simulink model "c00014M_harness"  (R2018a)
settings: Solver=ode3  StartTime=0.0  StopTime=10.0  RelTol=1e-3  EnableMultiTasking=on
undefined symbols (not defined in the file): b, DiscIntNeverNeededParam, J, K, L, PosMinimaW4, R, sigbuilder_block
(part 11 of 46)

== system c00014M_harness/M018/Cyber ==
  note: Sensors
  note: Inputs For Window1
  note: Inputs for Window 2
  note: Inputs for window 3
  note: Inputs for window 4
  note: Users
  note: Users
  note: Sensors
  note: Users
  note: Sensors
  note: Users
  note: Sensors
  note: USERS
      | ---------------------------------
      | 0: None
      | 1: Ventana Arriba
      | 2: Ventana hasta arriba
      | 3: Ventana abajo
      | 4: Ventana hasta abajo
  note: 1: SUBE
      | 0: PARADO
      | -1 BAJA
  note: D = Driver (W1)
      | P1 = Passenger 1 (W2)
      | P2 = Passenger 2 (W3)
      | P3 = Passenger 3 (W4)
      | O = Obstacle
      | C = Control
      | Pri = Prioritizer
      | LD = LockDriver
      | PosW = PositionWindow
      | WL = WindowLogic
      | OW = ObstacleWindow
      | CWXC = ControlWindowXCentralized
      | S = Sensor
      | L = Lock
      | WPos = WindowPosition
      | M = Memory
      | InW = InputWindow
      | WIn = WindowInput
  PosW1 : Inport
  PosW2 : Inport  Port=2
  PosW4 : Inport  Port=3
  DW1 : Inport  Port=4
  DW2 : Inport  Port=5
  DW4 : Inport  Port=6
  P1W2 : Inport  Port=7
  P3W4 : Inport  Port=8
  P1W4 : Inport  Port=9
  OW1 : Inport  Port=10
  OW2 : Inport  Port=11
  OW4 : Inport  Port=12
  LD : Inport  Port=13
  CW1C : Inport  Port=14
  CW2C : Inport  Port=15
  CW4C : Inport  Port=16
  Pri : Subsystem
  Pri3 : Subsystem
  Pri4 : Subsystem
  WL : Subsystem
  WL1 : Subsystem
  WL3 : Subsystem
  W1 : Outport
  W2 : Outport  Port=2
  W4 : Outport  Port=3
  wires:
  CW4C/1 -> Pri4/4(CW4C)
  CW2C/1 -> Pri/3(CW2C)
  CW1C/1 -> Pri3/2(CW1C)
  Pri3/1(User) -> WL/2(User)
  WL3/1(WindowLogicOutput) -> W4/1
  Pri4/1(User) -> WL3/2(User)
  OW4/1 -> WL3/3(OW)
  PosW4/1 -> WL3/1(WPos)
  P1W4/1 -> Pri4/3(P1)
  P3W4/1 -> Pri4/2(P)
  DW4/1 -> Pri4/1(D)
  WL1/1(WindowLogicOutput) -> W2/1
  OW2/1 -> WL1/3(OW)
  PosW2/1 -> WL1/1(WPos)
  P1W2/1 -> Pri/2(P)
  DW2/1 -> Pri/1(D)
  Pri/1(User) -> WL1/2(User)
  WL/1(WindowLogicOutput) -> W1/1
  DW1/1 -> Pri3/1(D)
  OW1/1 -> WL/3(OW)
  PosW1/1 -> WL/1(WPos)
  LD/1 -> WL1/4(L), WL3/4(L), WL/4(L)

== system c00014M_harness/M018/Physical ==
  InW1 : Inport
  InW2 : Inport  Port=2
  InW4 : Inport  Port=3
  W : Subsystem
  W5 : Subsystem
  W7 : Subsystem
  W1 : Outport
  W2 : Outport  Port=2
  W4 : Outport  Port=3
  wires:
  W7/1(WPos) -> W4/1
  W5/1(WPos) -> W2/1
  W/1(WPos) -> W1/1
  InW4/1 -> W7/1(WIn)
  InW2/1 -> W5/1(WIn)
  InW1/1 -> W/1(WIn)

== system c00014M_harness/M018/S1 ==
  PhyMeasure : Inport
  SensorOut : Outport
  wires:
  PhyMeasure/1 -> SensorOut/1

== system c00014M_harness/M018/S2 ==
  PhyMeasure : Inport
  SensorOut : Outport
  wires:
  PhyMeasure/1 -> SensorOut/1

== system c00014M_harness/M018/S4 ==
  PhyMeasure : Inport
  SensorOut : Outport
  wires:
  PhyMeasure/1 -> SensorOut/1

== system c00014M_harness/M019/Cyber ==
  note: Sensors
  note: Inputs For Window1
  note: Inputs for Window 2
  note: Inputs for window 3
  note: Inputs for window 4
  note: Users
  note: Users
  note: Sensors
  note: Users
  note: Sensors
  note: Users
  note: Sensors
  note: USERS
      | ---------------------------------
      | 0: None
      | 1: Ventana Arriba
      | 2: Ventana hasta arriba
      | 3: Ventana abajo
      | 4: Ventana hasta abajo
  note: 1: SUBE
      | 0: PARADO
      | -1 BAJA
  note: D = Driver (W1)
      | P1 = Passenger 1 (W2)
      | P2 = Passenger 2 (W3)
      | P3 = Passenger 3 (W4)
      | O = Obstacle
      | C = Control
      | Pri = Prioritizer
      | LD = LockDriver
      | PosW = PositionWindow
      | WL = WindowLogic
      | OW = ObstacleWindow
      | CWXC = ControlWindowXCentralized
      | S = Sensor
      | L = Lock
      | WPos = WindowPosition
      | M = Memory
      | InW = InputWindow
      | WIn = WindowInput
  PosW1 : Inport
  PosW2 : Inport  Port=2
  PosW4 : Inport  Port=3
  DW1 : Inport  Port=4
  DW2 : Inport  Port=5
  DW4 : Inport  Port=6
  P1W2 : Inport  Port=7
  P3W4 : Inport  Port=8
  P1W4 : Inport  Port=9
  OW1 : Inport  Port=10
  OW2 : Inport  Port=11
  OW4 : Inport  Port=12
  LD : Inport  Port=13
  CW1C : Inport  Port=14
  CW2C : Inport  Port=15
  CW4C : Inport  Port=16
  Pri : Subsystem
  Pri3 : Subsystem
  Pri4 : Subsystem
  WL : Subsystem
  WL1 : Subsystem
  WL3 : Subsystem
  W1 : Outport
  W2 : Outport  Port=2
  W4 : Outport  Port=3
  wires:
  CW4C/1 -> Pri4/4(CW4C)
  CW2C/1 -> Pri/3(CW2C)
  CW1C/1 -> Pri3/2(CW1C)
  Pri3/1(User) -> WL/2(User)
  WL3/1(WindowLogicOutput) -> W4/1
  Pri4/1(User) -> WL3/2(User)
  OW4/1 -> WL3/3(OW)
  PosW4/1 -> WL3/1(WPos)
  P1W4/1 -> Pri4/3(P1)
  P3W4/1 -> Pri4/2(P)
  DW4/1 -> Pri4/1(D)
  WL1/1(WindowLogicOutput) -> W2/1
  OW2/1 -> WL1/3(OW)
  PosW2/1 -> WL1/1(WPos)
  P1W2/1 -> Pri/2(P)
  DW2/1 -> Pri/1(D)
  Pri/1(User) -> WL1/2(User)
  WL/1(WindowLogicOutput) -> W1/1
  DW1/1 -> Pri3/1(D)
  OW1/1 -> WL/3(OW)
  PosW1/1 -> WL/1(WPos)
  LD/1 -> WL1/4(L), WL3/4(L), WL/4(L)

== system c00014M_harness/M019/Physical ==
  InW1 : Inport
  InW2 : Inport  Port=2
  InW4 : Inport  Port=3
  W : Subsystem
  W5 : Subsystem
  W7 : Subsystem
  W1 : Outport
  W2 : Outport  Port=2
  W4 : Outport  Port=3
  wires:
  W7/1(WPos) -> W4/1
  W5/1(WPos) -> W2/1
  W/1(WPos) -> W1/1
  InW4/1 -> W7/1(WIn)
  InW2/1 -> W5/1(WIn)
  InW1/1 -> W/1(WIn)

== system c00014M_harness/M019/S1 ==
  PhyMeasure : Inport
  SensorOut : Outport
  wires:
  PhyMeasure/1 -> SensorOut/1

== system c00014M_harness/M019/S2 ==
  PhyMeasure : Inport
  SensorOut : Outport
  wires:
  PhyMeasure/1 -> SensorOut/1

== system c00014M_harness/M019/S4 ==
  PhyMeasure : Inport
  SensorOut : Outport
  wires:
  PhyMeasure/1 -> SensorOut/1

== system c00014M_harness/M020/Cyber ==
  note: Sensors
  note: Inputs For Window1
  note: Inputs for Window 2
  note: Inputs for window 3
  note: Inputs for window 4
  note: Users
  note: Users
  note: Sensors
  note: Users
  note: Sensors
  note: Users
  note: Sensors
  note: USERS
      | ---------------------------------
      | 0: None
      | 1: Ventana Arriba
      | 2: Ventana hasta arriba
      | 3: Ventana abajo
      | 4: Ventana hasta abajo
  note: 1: SUBE
      | 0: PARADO
      | -1 BAJA
  note: D = Driver (W1)
      | P1 = Passenger 1 (W2)
      | P2 = Passenger 2 (W3)
      | P3 = Passenger 3 (W4)
      | O = Obstacle
      | C = Control
      | Pri = Prioritizer
      | LD = LockDriver
      | PosW = PositionWindow
      | WL = WindowLogic
      | OW = ObstacleWindow
      | CWXC = ControlWindowXCentralized
      | S = Sensor
      | L = Lock
      | WPos = WindowPosition
      | M = Memory
      | InW = InputWindow
      | WIn = WindowInput
  PosW1 : Inport
  PosW2 : Inport  Port=2
  PosW4 : Inport  Port=3
  DW1 : Inport  Port=4
  DW2 : Inport  Port=5
  DW4 : Inport  Port=6
  P1W2 : Inport  Port=7
  P3W4 : Inport  Port=8
  P1W4 : Inport  Port=9
  OW1 : Inport  Port=10
  OW2 : Inport  Port=11
  OW4 : Inport  Port=12
  LD : Inport  Port=13
  CW1C : Inport  Port=14
  CW2C : Inport  Port=15
  CW4C : Inport  Port=16
  Pri : Subsystem
  Pri3 : Subsystem
  Pri4 : Subsystem
  WL : Subsystem
  WL1 : Subsystem
  WL3 : Subsystem
  W1 : Outport
  W2 : Outport  Port=2
  W4 : Outport  Port=3
  wires:
  CW4C/1 -> Pri4/4(CW4C)
  CW2C/1 -> Pri/3(CW2C)
  CW1C/1 -> Pri3/2(CW1C)
  Pri3/1(User) -> WL/2(User)
  WL3/1(WindowLogicOutput) -> W4/1
  Pri4/1(User) -> WL3/2(User)
  OW4/1 -> WL3/3(OW)
  PosW4/1 -> WL3/1(WPos)
  P1W4/1 -> Pri4/3(P1)
  P3W4/1 -> Pri4/2(P)
  DW4/1 -> Pri4/1(D)
  WL1/1(WindowLogicOutput) -> W2/1
  OW2/1 -> WL1/3(OW)
  PosW2/1 -> WL1/1(WPos)
  P1W2/1 -> Pri/2(P)
  DW2/1 -> Pri/1(D)
  Pri/1(User) -> WL1/2(User)
  WL/1(WindowLogicOutput) -> W1/1
  DW1/1 -> Pri3/1(D)
  OW1/1 -> WL/3(OW)
  PosW1/1 -> WL/1(WPos)
  LD/1 -> WL1/4(L), WL3/4(L), WL/4(L)

== system c00014M_harness/M020/Physical ==
  InW1 : Inport
  InW2 : Inport  Port=2
  InW4 : Inport  Port=3
  W : Subsystem
  W5 : Subsystem
  W7 : Subsystem
  W1 : Outport
  W2 : Outport  Port=2
  W4 : Outport  Port=3
  wires:
  W7/1(WPos) -> W4/1
  W5/1(WPos) -> W2/1
  W/1(WPos) -> W1/1
  InW4/1 -> W7/1(WIn)
  InW2/1 -> W5/1(WIn)
  InW1/1 -> W/1(WIn)

== system c00014M_harness/M020/S1 ==
  PhyMeasure : Inport
  SensorOut : Outport
  wires:
  PhyMeasure/1 -> SensorOut/1

== system c00014M_harness/M020/S2 ==
  PhyMeasure : Inport
  SensorOut : Outport
  wires:
  PhyMeasure/1 -> SensorOut/1

== system c00014M_harness/M020/S4 ==
  PhyMeasure : Inport
  SensorOut : Outport
  wires:
  PhyMeasure/1 -> SensorOut/1

== system c00014M_harness/M022/Cyber ==
  note: Sensors
  note: Inputs For Window1
  note: Inputs for Window 2
  note: Inputs for window 3
  note: Inputs for window 4
  note: Users
  note: Users
  note: Sensors
  note: Users
  note: Sensors
  note: Users
  note: Sensors
  note: USERS
      | ---------------------------------
      | 0: None
      | 1: Ventana Arriba
      | 2: Ventana hasta arriba
      | 3: Ventana abajo
      | 4: Ventana hasta abajo
  note: 1: SUBE
      | 0: PARADO
      | -1 BAJA
  note: D = Driver (W1)
      | P1 = Passenger 1 (W2)
      | P2 = Passenger 2 (W3)
      | P3 = Passenger 3 (W4)
      | O = Obstacle
      | C = Control
      | Pri = Prioritizer
      | LD = LockDriver
      | PosW = PositionWindow
      | WL = WindowLogic
      | OW = ObstacleWindow
      | CWXC = ControlWindowXCentralized
      | S = Sensor
      | L = Lock
      | WPos = WindowPosition
      | M = Memory
      | InW = InputWindow
      | WIn = WindowInput
  PosW1 : Inport
  PosW2 : Inport  Port=2
  PosW4 : Inport  Port=3
  DW1 : Inport  Port=4
  DW2 : Inport  Port=5
  DW4 : Inport  Port=6
  P1W2 : Inport  Port=7
  P3W4 : Inport  Port=8
  P1W4 : Inport  Port=9
  OW1 : Inport  Port=10
  OW2 : Inport  Port=11
  OW4 : Inport  Port=12
  LD : Inport  Port=13
  CW1C : Inport  Port=14
  CW2C : Inport  Port=15
  CW4C : Inport  Port=16
  Pri : Subsystem
  Pri3 : Subsystem
  Pri4 : Subsystem
  WL : Subsystem
  WL1 : Subsystem
  WL3 : Subsystem
  W1 : Outport
  W2 : Outport  Port=2
  W4 : Outport  Port=3
  wires:
  CW4C/1 -> Pri4/4(CW4C)
  CW2C/1 -> Pri/3(CW2C)
  CW1C/1 -> Pri3/2(CW1C)
  Pri3/1(User) -> WL/2(User)
  WL3/1(WindowLogicOutput) -> W4/1
  Pri4/1(User) -> WL3/2(User)
  OW4/1 -> WL3/3(OW)
  PosW4/1 -> WL3/1(WPos)
  P1W4/1 -> Pri4/3(P1)
  P3W4/1 -> Pri4/2(P)
  DW4/1 -> Pri4/1(D)
  WL1/1(WindowLogicOutput) -> W2/1
  OW2/1 -> WL1/3(OW)
  PosW2/1 -> WL1/1(WPos)
  P1W2/1 -> Pri/2(P)
  DW2/1 -> Pri/1(D)
  Pri/1(User) -> WL1/2(User)
  WL/1(WindowLogicOutput) -> W1/1
  DW1/1 -> Pri3/1(D)
  OW1/1 -> WL/3(OW)
  PosW1/1 -> WL/1(WPos)
  LD/1 -> WL1/4(L), WL3/4(L), WL/4(L)

== system c00014M_harness/M022/Physical ==
  InW1 : Inport
  InW2 : Inport  Port=2
  InW4 : Inport  Port=3
  W : Subsystem
  W5 : Subsystem
  W7 : Subsystem
  W1 : Outport
  W2 : Outport  Port=2
  W4 : Outport  Port=3
  wires:
  W7/1(WPos) -> W4/1
  W5/1(WPos) -> W2/1
  W/1(WPos) -> W1/1
  InW4/1 -> W7/1(WIn)
  InW2/1 -> W5/1(WIn)
  InW1/1 -> W/1(WIn)

== system c00014M_harness/M022/S1 ==
  PhyMeasure : Inport
  SensorOut : Outport
  wires:
  PhyMeasure/1 -> SensorOut/1

== system c00014M_harness/M022/S2 ==
  PhyMeasure : Inport
  SensorOut : Outport
  wires:
  PhyMeasure/1 -> SensorOut/1

== system c00014M_harness/M022/S4 ==
  PhyMeasure : Inport
  SensorOut : Outport
  wires:
  PhyMeasure/1 -> SensorOut/1

== system c00014M_harness/M023/Cyber ==
  note: Sensors
  note: Inputs For Window1
  note: Inputs for Window 2
  note: Inputs for window 3
  note: Inputs for window 4
  note: Users
  note: Users
  note: Sensors
  note: Users
  note: Sensors
  note: Users
  note: Sensors
  note: USERS
      | ---------------------------------
      | 0: None
      | 1: Ventana Arriba
      | 2: Ventana hasta arriba
      | 3: Ventana abajo
      | 4: Ventana hasta abajo
  note: 1: SUBE
      | 0: PARADO
      | -1 BAJA
  note: D = Driver (W1)
      | P1 = Passenger 1 (W2)
      | P2 = Passenger 2 (W3)
      | P3 = Passenger 3 (W4)
      | O = Obstacle
      | C = Control
      | Pri = Prioritizer
      | LD = LockDriver
      | PosW = PositionWindow
      | WL = WindowLogic
      | OW = ObstacleWindow
      | CWXC = ControlWindowXCentralized
      | S = Sensor
      | L = Lock
      | WPos = WindowPosition
      | M = Memory
      | InW = InputWindow
      | WIn = WindowInput
  PosW1 : Inport
  PosW2 : Inport  Port=2
  PosW4 : Inport  Port=3
  DW1 : Inport  Port=4
  DW2 : Inport  Port=5
  DW4 : Inport  Port=6
  P1W2 : Inport  Port=7
  P3W4 : Inport  Port=8
  P1W4 : Inport  Port=9
  OW1 : Inport  Port=10
  OW2 : Inport  Port=11
  OW4 : Inport  Port=12
  LD : Inport  Port=13
  CW1C : Inport  Port=14
  CW2C : Inport  Port=15
  CW4C : Inport  Port=16
  Pri : Subsystem
  Pri3 : Subsystem
  Pri4 : Subsystem
  WL : Subsystem
  WL1 : Subsystem
  WL3 : Subsystem
  W1 : Outport
  W2 : Outport  Port=2
  W4 : Outport  Port=3
  wires:
  CW4C/1 -> Pri4/4(CW4C)
  CW2C/1 -> Pri/3(CW2C)
  CW1C/1 -> Pri3/2(CW1C)
  Pri3/1(User) -> WL/2(User)
  WL3/1(WindowLogicOutput) -> W4/1
  Pri4/1(User) -> WL3/2(User)
  OW4/1 -> WL3/3(OW)
  PosW4/1 -> WL3/1(WPos)
  P1W4/1 -> Pri4/3(P1)
  P3W4/1 -> Pri4/2(P)
  DW4/1 -> Pri4/1(D)
  WL1/1(WindowLogicOutput) -> W2/1
  OW2/1 -> WL1/3(OW)
  PosW2/1 -> WL1/1(WPos)
  P1W2/1 -> Pri/2(P)
  DW2/1 -> Pri/1(D)
  Pri/1(User) -> WL1/2(User)
  WL/1(WindowLogicOutput) -> W1/1
  DW1/1 -> Pri3/1(D)
  OW1/1 -> WL/3(OW)
  PosW1/1 -> WL/1(WPos)
  LD/1 -> WL1/4(L), WL3/4(L), WL/4(L)

== system c00014M_harness/M023/Physical ==
  InW1 : Inport
  InW2 : Inport  Port=2
  InW4 : Inport  Port=3
  W : Subsystem
  W5 : Subsystem
  W7 : Subsystem
  W1 : Outport
  W2 : Outport  Port=2
  W4 : Outport  Port=3
  wires:
  W7/1(WPos) -> W4/1
  W5/1(WPos) -> W2/1
  W/1(WPos) -> W1/1
  InW4/1 -> W7/1(WIn)
  InW2/1 -> W5/1(WIn)
  InW1/1 -> W/1(WIn)

== system c00014M_harness/M023/S1 ==
  PhyMeasure : Inport
  SensorOut : Outport
  wires:
  PhyMeasure/1 -> SensorOut/1

== system c00014M_harness/M023/S2 ==
  PhyMeasure : Inport
  SensorOut : Outport
  wires:
  PhyMeasure/1 -> SensorOut/1

== system c00014M_harness/M023/S4 ==
  PhyMeasure : Inport
  SensorOut : Outport
  wires:
  PhyMeasure/1 -> SensorOut/1

== system c00014M_harness/M024/Cyber ==
  note: Sensors
  note: Inputs For Window1
  note: Inputs for Window 2
  note: Inputs for window 3
  note: Inputs for window 4
  note: Users
  note: Users
  note: Sensors
  note: Users
  note: Sensors
  note: Users
  note: Sensors
  note: USERS
      | ---------------------------------
      | 0: None
      | 1: Ventana Arriba
      | 2: Ventana hasta arriba
      | 3: Ventana abajo
      | 4: Ventana hasta abajo
  note: 1: SUBE
      | 0: PARADO
      | -1 BAJA
  note: D = Driver (W1)
      | P1 = Passenger 1 (W2)
      | P2 = Passenger 2 (W3)
      | P3 = Passenger 3 (W4)
      | O = Obstacle
      | C = Control
      | Pri = Prioritizer
      | LD = LockDriver
      | PosW = PositionWindow
      | WL = WindowLogic
      | OW = ObstacleWindow
      | CWXC = ControlWindowXCentralized
      | S = Sensor
      | L = Lock
      | WPos = WindowPosition
      | M = Memory
      | InW = InputWindow
      | WIn = WindowInput
  PosW1 : Inport
  PosW2 : Inport  Port=2
  PosW4 : Inport  Port=3
  DW1 : Inport  Port=4
  DW2 : Inport  Port=5
  DW4 : Inport  Port=6
  P1W2 : Inport  Port=7
  P3W4 : Inport  Port=8
  P1W4 : Inport  Port=9
  OW1 : Inport  Port=10
  OW2 : Inport  Port=11
  OW4 : Inport  Port=12
  LD : Inport  Port=13
  CW1C : Inport  Port=14
  CW2C : Inport  Port=15
  CW4C : Inport  Port=16
  Pri : Subsystem
  Pri3 : Subsystem
  Pri4 : Subsystem
  WL : Subsystem
  WL1 : Subsystem
  WL3 : Subsystem
  W1 : Outport
  W2 : Outport  Port=2
  W4 : Outport  Port=3
  wires:
  CW4C/1 -> Pri4/4(CW4C)
  CW2C/1 -> Pri/3(CW2C)
  CW1C/1 -> Pri3/2(CW1C)
  Pri3/1(User) -> WL/2(User)
  WL3/1(WindowLogicOutput) -> W4/1
  Pri4/1(User) -> WL3/2(User)
  OW4/1 -> WL3/3(OW)
  PosW4/1 -> WL3/1(WPos)
  P1W4/1 -> Pri4/3(P1)
  P3W4/1 -> Pri4/2(P)
  DW4/1 -> Pri4/1(D)
  WL1/1(WindowLogicOutput) -> W2/1
  OW2/1 -> WL1/3(OW)
  PosW2/1 -> WL1/1(WPos)
  P1W2/1 -> Pri/2(P)
  DW2/1 -> Pri/1(D)
  Pri/1(User) -> WL1/2(User)
  WL/1(WindowLogicOutput) -> W1/1
  DW1/1 -> Pri3/1(D)
  OW1/1 -> WL/3(OW)
  PosW1/1 -> WL/1(WPos)
  LD/1 -> WL1/4(L), WL3/4(L), WL/4(L)

== system c00014M_harness/M024/Physical ==
  InW1 : Inport
  InW2 : Inport  Port=2
  InW4 : Inport  Port=3
  W : Subsystem
  W5 : Subsystem
  W7 : Subsystem
  W1 : Outport
  W2 : Outport  Port=2
  W4 : Outport  Port=3
  wires:
  W7/1(WPos) -> W4/1
  W5/1(WPos) -> W2/1
  W/1(WPos) -> W1/1
  InW4/1 -> W7/1(WIn)
  InW2/1 -> W5/1(WIn)
  InW1/1 -> W/1(WIn)

== system c00014M_harness/M024/S1 ==
  PhyMeasure : Inport
  SensorOut : Outport
  wires:
  PhyMeasure/1 -> SensorOut/1

== system c00014M_harness/M024/S2 ==
  PhyMeasure : Inport
  SensorOut : Outport
  wires:
  PhyMeasure/1 -> SensorOut/1

== system c00014M_harness/M024/S4 ==
  PhyMeasure : Inport
  SensorOut : Outport
  wires:
  PhyMeasure/1 -> SensorOut/1

== system c00014M_harness/M026/Cyber ==
  note: Sensors
  note: Inputs For Window1
  note: Inputs for Window 2
  note: Inputs for window 3
  note: Inputs for window 4
  note: Users
  note: Users
  note: Sensors
  note: Users
  note: Sensors
  note: Users
  note: Sensors
  note: USERS
      | ---------------------------------
      | 0: None
      | 1: Ventana Arriba
      | 2: Ventana hasta arriba
      | 3: Ventana abajo
      | 4: Ventana hasta abajo
  note: 1: SUBE
      | 0: PARADO
      | -1 BAJA
  note: D = Driver (W1)
      | P1 = Passenger 1 (W2)
      | P2 = Passenger 2 (W3)
      | P3 = Passenger 3 (W4)
      | O = Obstacle
      | C = Control
      | Pri = Prioritizer
      | LD = LockDriver
      | PosW = PositionWindow
      | WL = WindowLogic
      | OW = ObstacleWindow
      | CWXC = ControlWindowXCentralized
      | S = Sensor
      | L = Lock
      | WPos = WindowPosition
      | M = Memory
      | InW = InputWindow
      | WIn = WindowInput
  PosW1 : Inport
  PosW2 : Inport  Port=2
  PosW4 : Inport  Port=3
  DW1 : Inport  Port=4
  DW2 : Inport  Port=5
  DW4 : Inport  Port=6
  P1W2 : Inport  Port=7
  P3W4 : Inport  Port=8
  P1W4 : Inport  Port=9
  OW1 : Inport  Port=10
  OW2 : Inport  Port=11
  OW4 : Inport  Port=12
  LD : Inport  Port=13
  CW1C : Inport  Port=14
  CW2C : Inport  Port=15
  CW4C : Inport  Port=16
  Pri : Subsystem
  Pri3 : Subsystem
  Pri4 : Subsystem
  WL : Subsystem
  WL1 : Subsystem
  WL3 : Subsystem
  W1 : Outport
  W2 : Outport  Port=2
  W4 : Outport  Port=3
  wires:
  CW4C/1 -> Pri4/4(CW4C)
  CW2C/1 -> Pri/3(CW2C)
  CW1C/1 -> Pri3/2(CW1C)
  Pri3/1(User) -> WL/2(User)
  WL3/1(WindowLogicOutput) -> W4/1
  Pri4/1(User) -> WL3/2(User)
  OW4/1 -> WL3/3(OW)
  PosW4/1 -> WL3/1(WPos)
  P1W4/1 -> Pri4/3(P1)
  P3W4/1 -> Pri4/2(P)
  DW4/1 -> Pri4/1(D)
  WL1/1(WindowLogicOutput) -> W2/1
  OW2/1 -> WL1/3(OW)
  PosW2/1 -> WL1/1(WPos)
  P1W2/1 -> Pri/2(P)
  DW2/1 -> Pri/1(D)
  Pri/1(User) -> WL1/2(User)
  WL/1(WindowLogicOutput) -> W1/1
  DW1/1 -> Pri3/1(D)
  OW1/1 -> WL/3(OW)
  PosW1/1 -> WL/1(WPos)
  LD/1 -> WL1/4(L), WL3/4(L), WL/4(L)

== system c00014M_harness/M026/Physical ==
  InW1 : Inport
  InW2 : Inport  Port=2
  InW4 : Inport  Port=3
  W : Subsystem
  W5 : Subsystem
  W7 : Subsystem
  W1 : Outport
  W2 : Outport  Port=2
  W4 : Outport  Port=3
  wires:
  W7/1(WPos) -> W4/1
  W5/1(WPos) -> W2/1
  W/1(WPos) -> W1/1
  InW4/1 -> W7/1(WIn)
  InW2/1 -> W5/1(WIn)
  InW1/1 -> W/1(WIn)

== system c00014M_harness/M026/S1 ==
  PhyMeasure : Inport
  SensorOut : Outport
  wires:
  PhyMeasure/1 -> SensorOut/1

== system c00014M_harness/M026/S2 ==
  PhyMeasure : Inport
  SensorOut : Outport
  wires:
  PhyMeasure/1 -> SensorOut/1

== system c00014M_harness/M026/S4 ==
  PhyMeasure : Inport
  SensorOut : Outport
  wires:
  PhyMeasure/1 -> SensorOut/1

== system c00014M_harness/M027/Cyber ==
  note: Sensors
  note: Inputs For Window1
  note: Inputs for Window 2
  note: Inputs for window 3
  note: Inputs for window 4
  note: Users
  note: Users
  note: Sensors
  note: Users
  note: Sensors
  note: Users
  note: Sensors
  note: USERS
      | ---------------------------------
      | 0: None
      | 1: Ventana Arriba
      | 2: Ventana hasta arriba
      | 3: Ventana abajo
      | 4: Ventana hasta abajo
  note: 1: SUBE
      | 0: PARADO
      | -1 BAJA
  note: D = Driver (W1)
      | P1 = Passenger 1 (W2)
      | P2 = Passenger 2 (W3)
      | P3 = Passenger 3 (W4)
      | O = Obstacle
      | C = Control
      | Pri = Prioritizer
      | LD = LockDriver
      | PosW = PositionWindow
      | WL = WindowLogic
      | OW = ObstacleWindow
      | CWXC = ControlWindowXCentralized
      | S = Sensor
      | L = Lock
      | WPos = WindowPosition
      | M = Memory
      | InW = InputWindow
      | WIn = WindowInput
  PosW1 : Inport
  PosW2 : Inport  Port=2
  PosW4 : Inport  Port=3
  DW1 : Inport  Port=4
  DW2 : Inport  Port=5
  DW4 : Inport  Port=6
  P1W2 : Inport  Port=7
  P3W4 : Inport  Port=8
  P1W4 : Inport  Port=9
  OW1 : Inport  Port=10
  OW2 : Inport  Port=11
  OW4 : Inport  Port=12
  LD : Inport  Port=13
  CW1C : Inport  Port=14
  CW2C : Inport  Port=15
  CW4C : Inport  Port=16
  Pri : Subsystem
  Pri3 : Subsystem
  Pri4 : Subsystem
  WL : Subsystem
  WL1 : Subsystem
  WL3 : Subsystem
  W1 : Outport
  W2 : Outport  Port=2
  W4 : Outport  Port=3
  wires:
  CW4C/1 -> Pri4/4(CW4C)
  CW2C/1 -> Pri/3(CW2C)
  CW1C/1 -> Pri3/2(CW1C)
  Pri3/1(User) -> WL/2(User)
  WL3/1(WindowLogicOutput) -> W4/1
  Pri4/1(User) -> WL3/2(User)
  OW4/1 -> WL3/3(OW)
  PosW4/1 -> WL3/1(WPos)
  P1W4/1 -> Pri4/3(P1)
  P3W4/1 -> Pri4/2(P)
  DW4/1 -> Pri4/1(D)
  WL1/1(WindowLogicOutput) -> W2/1
  OW2/1 -> WL1/3(OW)
  PosW2/1 -> WL1/1(WPos)
  P1W2/1 -> Pri/2(P)
  DW2/1 -> Pri/1(D)
  Pri/1(User) -> WL1/2(User)
  WL/1(WindowLogicOutput) -> W1/1
  DW1/1 -> Pri3/1(D)
  OW1/1 -> WL/3(OW)
  PosW1/1 -> WL/1(WPos)
  LD/1 -> WL1/4(L), WL3/4(L), WL/4(L)

== system c00014M_harness/M027/Physical ==
  InW1 : Inport
  InW2 : Inport  Port=2
  InW4 : Inport  Port=3
  W : Subsystem
  W5 : Subsystem
  W7 : Subsystem
  W1 : Outport
  W2 : Outport  Port=2
  W4 : Outport  Port=3
  wires:
  W7/1(WPos) -> W4/1
  W5/1(WPos) -> W2/1
  W/1(WPos) -> W1/1
  InW4/1 -> W7/1(WIn)
  InW2/1 -> W5/1(WIn)
  InW1/1 -> W/1(WIn)

== system c00014M_harness/M027/S1 ==
  PhyMeasure : Inport
  SensorOut : Outport
  wires:
  PhyMeasure/1 -> SensorOut/1

== system c00014M_harness/M027/S2 ==
  PhyMeasure : Inport
  SensorOut : Outport
  wires:
  PhyMeasure/1 -> SensorOut/1

== system c00014M_harness/M027/S4 ==
  PhyMeasure : Inport
  SensorOut : Outport
  wires:
  PhyMeasure/1 -> SensorOut/1

== system c00014M_harness/M028/Cyber ==
  note: Sensors
  note: Inputs For Window1
  note: Inputs for Window 2
  note: Inputs for window 3
  note: Inputs for window 4
  note: Users
  note: Users
  note: Sensors
  note: Users
  note: Sensors
  note: Users
  note: Sensors
  note: USERS
      | ---------------------------------
      | 0: None
      | 1: Ventana Arriba
      | 2: Ventana hasta arriba
      | 3: Ventana abajo
      | 4: Ventana hasta abajo
  note: 1: SUBE
      | 0: PARADO
      | -1 BAJA
  note: D = Driver (W1)
      | P1 = Passenger 1 (W2)
      | P2 = Passenger 2 (W3)
      | P3 = Passenger 3 (W4)
      | O = Obstacle
      | C = Control
      | Pri = Prioritizer
      | LD = LockDriver
      | PosW = PositionWindow
      | WL = WindowLogic
      | OW = ObstacleWindow
      | CWXC = ControlWindowXCentralized
      | S = Sensor
      | L = Lock
      | WPos = WindowPosition
      | M = Memory
      | InW = InputWindow
      | WIn = WindowInput
  PosW1 : Inport
  PosW2 : Inport  Port=2
  PosW4 : Inport  Port=3
  DW1 : Inport  Port=4
  DW2 : Inport  Port=5
  DW4 : Inport  Port=6
  P1W2 : Inport  Port=7
  P3W4 : Inport  Port=8
  P1W4 : Inport  Port=9
  OW1 : Inport  Port=10
  OW2 : Inport  Port=11
  OW4 : Inport  Port=12
  LD : Inport  Port=13
  CW1C : Inport  Port=14
  CW2C : Inport  Port=15
  CW4C : Inport  Port=16
  Pri : Subsystem
  Pri3 : Subsystem
  Pri4 : Subsystem
  WL : Subsystem
  WL1 : Subsystem
  WL3 : Subsystem
  W1 : Outport
  W2 : Outport  Port=2
  W4 : Outport  Port=3
  wires:
  CW4C/1 -> Pri4/4(CW4C)
  CW2C/1 -> Pri/3(CW2C)
  CW1C/1 -> Pri3/2(CW1C)
  Pri3/1(User) -> WL/2(User)
  WL3/1(WindowLogicOutput) -> W4/1
  Pri4/1(User) -> WL3/2(User)
  OW4/1 -> WL3/3(OW)
  PosW4/1 -> WL3/1(WPos)
  P1W4/1 -> Pri4/3(P1)
  P3W4/1 -> Pri4/2(P)
  DW4/1 -> Pri4/1(D)
  WL1/1(WindowLogicOutput) -> W2/1
  OW2/1 -> WL1/3(OW)
  PosW2/1 -> WL1/1(WPos)
  P1W2/1 -> Pri/2(P)
  DW2/1 -> Pri/1(D)
  Pri/1(User) -> WL1/2(User)
  WL/1(WindowLogicOutput) -> W1/1
  DW1/1 -> Pri3/1(D)
  OW1/1 -> WL/3(OW)
  PosW1/1 -> WL/1(WPos)
  LD/1 -> WL1/4(L), WL3/4(L), WL/4(L)

== system c00014M_harness/M028/Physical ==
  InW1 : Inport
  InW2 : Inport  Port=2
  InW4 : Inport  Port=3
  W : Subsystem
  W5 : Subsystem
  W7 : Subsystem
  W1 : Outport
  W2 : Outport  Port=2
  W4 : Outport  Port=3
  wires:
  W7/1(WPos) -> W4/1
  W5/1(WPos) -> W2/1
  W/1(WPos) -> W1/1
  InW4/1 -> W7/1(WIn)
  InW2/1 -> W5/1(WIn)
  InW1/1 -> W/1(WIn)

== system c00014M_harness/M028/S1 ==
  PhyMeasure : Inport
  SensorOut : Outport
  wires:
  PhyMeasure/1 -> SensorOut/1

== system c00014M_harness/M028/S2 ==
  PhyMeasure : Inport
  SensorOut : Outport
  wires:
  PhyMeasure/1 -> SensorOut/1

== system c00014M_harness/M028/S4 ==
  PhyMeasure : Inport
  SensorOut : Outport
  wires:
  PhyMeasure/1 -> SensorOut/1

== system c00014M_harness/M030/Cyber ==
  note: Sensors
  note: Inputs For Window1
  note: Inputs for Window 2
  note: Inputs for window 3
  note: Inputs for window 4
  note: Users
  note: Users
  note: Sensors
  note: Users
  note: Sensors
  note: Users
  note: Sensors
  note: USERS
      | ---------------------------------
      | 0: None
      | 1: Ventana Arriba
      | 2: Ventana hasta arriba
      | 3: Ventana abajo
      | 4: Ventana hasta abajo
  note: 1: SUBE
      | 0: PARADO
      | -1 BAJA
  note: D = Driver (W1)
      | P1 = Passenger 1 (W2)
      | P2 = Passenger 2 (W3)
      | P3 = Passenger 3 (W4)
      | O = Obstacle
      | C = Control
      | Pri = Prioritizer
      | LD = LockDriver
      | PosW = PositionWindow
      | WL = WindowLogic
      | OW = ObstacleWindow
      | CWXC = ControlWindowXCentralized
      | S = Sensor
      | L = Lock
      | WPos = WindowPosition
      | M = Memory
      | InW = InputWindow
      | WIn = WindowInput
  PosW1 : Inport
  PosW2 : Inport  Port=2
  PosW4 : Inport  Port=3
  DW1 : Inport  Port=4
  DW2 : Inport  Port=5
  DW4 : Inport  Port=6
  P1W2 : Inport  Port=7
  P3W4 : Inport  Port=8
  P1W4 : Inport  Port=9
  OW1 : Inport  Port=10
  OW2 : Inport  Port=11
  OW4 : Inport  Port=12
  LD : Inport  Port=13
  CW1C : Inport  Port=14
  CW2C : Inport  Port=15
  CW4C : Inport  Port=16
  Pri : Subsystem
  Pri3 : Subsystem
  Pri4 : Subsystem
  WL : Subsystem
  WL1 : Subsystem
  WL3 : Subsystem
  W1 : Outport
  W2 : Outport  Port=2
  W4 : Outport  Port=3
  wires:
  CW4C/1 -> Pri4/4(CW4C)
  CW2C/1 -> Pri/3(CW2C)
  CW1C/1 -> Pri3/2(CW1C)
  Pri3/1(User) -> WL/2(User)
  WL3/1(WindowLogicOutput) -> W4/1
  Pri4/1(User) -> WL3/2(User)
  OW4/1 -> WL3/3(OW)
  PosW4/1 -> WL3/1(WPos)
  P1W4/1 -> Pri4/3(P1)
  P3W4/1 -> Pri4/2(P)
  DW4/1 -> Pri4/1(D)
  WL1/1(WindowLogicOutput) -> W2/1
  OW2/1 -> WL1/3(OW)
  PosW2/1 -> WL1/1(WPos)
  P1W2/1 -> Pri/2(P)
  DW2/1 -> Pri/1(D)
  Pri/1(User) -> WL1/2(User)
  WL/1(WindowLogicOutput) -> W1/1
  DW1/1 -> Pri3/1(D)
  OW1/1 -> WL/3(OW)
  PosW1/1 -> WL/1(WPos)
  LD/1 -> WL1/4(L), WL3/4(L), WL/4(L)

== system c00014M_harness/M030/Physical ==
  InW1 : Inport
  InW2 : Inport  Port=2
  InW4 : Inport  Port=3
  W : Subsystem
  W5 : Subsystem
  W7 : Subsystem
  W1 : Outport
  W2 : Outport  Port=2
  W4 : Outport  Port=3
  wires:
  W7/1(WPos) -> W4/1
  W5/1(WPos) -> W2/1
  W/1(WPos) -> W1/1
  InW4/1 -> W7/1(WIn)
  InW2/1 -> W5/1(WIn)
  InW1/1 -> W/1(WIn)

== system c00014M_harness/M030/S1 ==
  PhyMeasure : Inport
  SensorOut : Outport
  wires:
  PhyMeasure/1 -> SensorOut/1

== system c00014M_harness/M030/S2 ==
  PhyMeasure : Inport
  SensorOut : Outport
  wires:
  PhyMeasure/1 -> SensorOut/1

== system c00014M_harness/M030/S4 ==
  PhyMeasure : Inport
  SensorOut : Outport
  wires:
  PhyMeasure/1 -> SensorOut/1

== system c00014M_harness/M031/Cyber ==
  note: Sensors
  note: Inputs For Window1
  note: Inputs for Window 2
  note: Inputs for window 3
  note: Inputs for window 4
  note: Users
  note: Users
  note: Sensors
  note: Users
  note: Sensors
  note: Users
  note: Sensors
  note: USERS
      | ---------------------------------
      | 0: None
      | 1: Ventana Arriba
      | 2: Ventana hasta arriba
      | 3: Ventana abajo
      | 4: Ventana hasta abajo
  note: 1: SUBE
      | 0: PARADO
      | -1 BAJA
  note: D = Driver (W1)
      | P1 = Passenger 1 (W2)
      | P2 = Passenger 2 (W3)
      | P3 = Passenger 3 (W4)
      | O = Obstacle
      | C = Control
      | Pri = Prioritizer
      | LD = LockDriver
      | PosW = PositionWindow
      | WL = WindowLogic
      | OW = ObstacleWindow
      | CWXC = ControlWindowXCentralized
      | S = Sensor
      | L = Lock
      | WPos = WindowPosition
      | M = Memory
      | InW = InputWindow
      | WIn = WindowInput
  PosW1 : Inport
  PosW2 : Inport  Port=2
  PosW4 : Inport  Port=3
  DW1 : Inport  Port=4
  DW2 : Inport  Port=5
  DW4 : Inport  Port=6
  P1W2 : Inport  Port=7
  P3W4 : Inport  Port=8
  P1W4 : Inport  Port=9
  OW1 : Inport  Port=10
  OW2 : Inport  Port=11
  OW4 : Inport  Port=12
  LD : Inport  Port=13
  CW1C : Inport  Port=14
  CW2C : Inport  Port=15
  CW4C : Inport  Port=16
  Pri : Subsystem
  Pri3 : Subsystem
  Pri4 : Subsystem
  WL : Subsystem
  WL1 : Subsystem
  WL3 : Subsystem
  W1 : Outport
  W2 : Outport  Port=2
  W4 : Outport  Port=3
  wires:
  CW4C/1 -> Pri4/4(CW4C)
  CW2C/1 -> Pri/3(CW2C)
  CW1C/1 -> Pri3/2(CW1C)
  Pri3/1(User) -> WL/2(User)
  WL3/1(WindowLogicOutput) -> W4/1
  Pri4/1(User) -> WL3/2(User)
  OW4/1 -> WL3/3(OW)
  PosW4/1 -> WL3/1(WPos)
  P1W4/1 -> Pri4/3(P1)
  P3W4/1 -> Pri4/2(P)
  DW4/1 -> Pri4/1(D)
  WL1/1(WindowLogicOutput) -> W2/1
  OW2/1 -> WL1/3(OW)
  PosW2/1 -> WL1/1(WPos)
  P1W2/1 -> Pri/2(P)
  DW2/1 -> Pri/1(D)
  Pri/1(User) -> WL1/2(User)
  WL/1(WindowLogicOutput) -> W1/1
  DW1/1 -> Pri3/1(D)
  OW1/1 -> WL/3(OW)
  PosW1/1 -> WL/1(WPos)
  LD/1 -> WL1/4(L), WL3/4(L), WL/4(L)

== system c00014M_harness/M031/Physical ==
  InW1 : Inport
  InW2 : Inport  Port=2
  InW4 : Inport  Port=3
  W : Subsystem
  W5 : Subsystem
  W7 : Subsystem
  W1 : Outport
  W2 : Outport  Port=2
  W4 : Outport  Port=3
  wires:
  W7/1(WPos) -> W4/1
  W5/1(WPos) -> W2/1
  W/1(WPos) -> W1/1
  InW4/1 -> W7/1(WIn)
  InW2/1 -> W5/1(WIn)
  InW1/1 -> W/1(WIn)

== system c00014M_harness/M031/S1 ==
  PhyMeasure : Inport
  SensorOut : Outport
  wires:
  PhyMeasure/1 -> SensorOut/1

== system c00014M_harness/M031/S2 ==
  PhyMeasure : Inport
  SensorOut : Outport
  wires:
  PhyMeasure/1 -> SensorOut/1

== system c00014M_harness/M031/S4 ==
  PhyMeasure : Inport
  SensorOut : Outport
  wires:
  PhyMeasure/1 -> SensorOut/1

== system c00014M_harness/M032/Cyber ==
  note: Sensors
  note: Inputs For Window1
  note: Inputs for Window 2
  note: Inputs for window 3
  note: Inputs for window 4
  note: Users
  note: Users
  note: Sensors
  note: Users
  note: Sensors
  note: Users
  note: Sensors
  note: USERS
      | ---------------------------------
      | 0: None
      | 1: Ventana Arriba
      | 2: Ventana hasta arriba
      | 3: Ventana abajo
      | 4: Ventana hasta abajo
  note: 1: SUBE
      | 0: PARADO
      | -1 BAJA
  note: D = Driver (W1)
      | P1 = Passenger 1 (W2)
      | P2 = Passenger 2 (W3)
      | P3 = Passenger 3 (W4)
      | O = Obstacle
      | C = Control
      | Pri = Prioritizer
      | LD = LockDriver
      | PosW = PositionWindow
      | WL = WindowLogic
      | OW = ObstacleWindow
      | CWXC = ControlWindowXCentralized
      | S = Sensor
      | L = Lock
      | WPos = WindowPosition
      | M = Memory
      | InW = InputWindow
      | WIn = WindowInput
  PosW1 : Inport
  PosW2 : Inport  Port=2
  PosW4 : Inport  Port=3
  DW1 : Inport  Port=4
  DW2 : Inport  Port=5
  DW4 : Inport  Port=6
  P1W2 : Inport  Port=7
  P3W4 : Inport  Port=8
  P1W4 : Inport  Port=9
  OW1 : Inport  Port=10
  OW2 : Inport  Port=11
  OW4 : Inport  Port=12
  LD : Inport  Port=13
  CW1C : Inport  Port=14
  CW2C : Inport  Port=15
  CW4C : Inport  Port=16
  Pri : Subsystem
  Pri3 : Subsystem
  Pri4 : Subsystem
  WL : Subsystem
  WL1 : Subsystem
  WL3 : Subsystem
  W1 : Outport
  W2 : Outport  Port=2
  W4 : Outport  Port=3
  wires:
  CW4C/1 -> Pri4/4(CW4C)
  CW2C/1 -> Pri/3(CW2C)
  CW1C/1 -> Pri3/2(CW1C)
  Pri3/1(User) -> WL/2(User)
  WL3/1(WindowLogicOutput) -> W4/1
  Pri4/1(User) -> WL3/2(User)
  OW4/1 -> WL3/3(OW)
  PosW4/1 -> WL3/1(WPos)
  P1W4/1 -> Pri4/3(P1)
  P3W4/1 -> Pri4/2(P)
  DW4/1 -> Pri4/1(D)
  WL1/1(WindowLogicOutput) -> W2/1
  OW2/1 -> WL1/3(OW)
  PosW2/1 -> WL1/1(WPos)
  P1W2/1 -> Pri/2(P)
  DW2/1 -> Pri/1(D)
  Pri/1(User) -> WL1/2(User)
  WL/1(WindowLogicOutput) -> W1/1
  DW1/1 -> Pri3/1(D)
  OW1/1 -> WL/3(OW)
  PosW1/1 -> WL/1(WPos)
  LD/1 -> WL1/4(L), WL3/4(L), WL/4(L)

== system c00014M_harness/M032/Physical ==
  InW1 : Inport
  InW2 : Inport  Port=2
  InW4 : Inport  Port=3
  W : Subsystem
  W5 : Subsystem
  W7 : Subsystem
  W1 : Outport
  W2 : Outport  Port=2
  W4 : Outport  Port=3
  wires:
  W7/1(WPos) -> W4/1
  W5/1(WPos) -> W2/1
  W/1(WPos) -> W1/1
  InW4/1 -> W7/1(WIn)
  InW2/1 -> W5/1(WIn)
  InW1/1 -> W/1(WIn)

== system c00014M_harness/M032/S1 ==
  PhyMeasure : Inport
  SensorOut : Outport
  wires:
  PhyMeasure/1 -> SensorOut/1

== system c00014M_harness/M032/S2 ==
  PhyMeasure : Inport
  SensorOut : Outport
  wires:
  PhyMeasure/1 -> SensorOut/1

== system c00014M_harness/M032/S4 ==
  PhyMeasure : Inport
  SensorOut : Outport
  wires:
  PhyMeasure/1 -> SensorOut/1

== system c00014M_harness/M034/Cyber ==
  note: Sensors
  note: Inputs For Window1
  note: Inputs for Window 2
  note: Inputs for window 3
  note: Inputs for window 4
  note: Users
  note: Users
  note: Sensors
  note: Users
  note: Sensors
  note: Users
  note: Sensors
  note: USERS
      | ---------------------------------
      | 0: None
      | 1: Ventana Arriba
      | 2: Ventana hasta arriba
      | 3: Ventana abajo
      | 4: Ventana hasta abajo
  note: 1: SUBE
      | 0: PARADO
      | -1 BAJA
  note: D = Driver (W1)
      | P1 = Passenger 1 (W2)
      | P2 = Passenger 2 (W3)
      | P3 = Passenger 3 (W4)
      | O = Obstacle
      | C = Control
      | Pri = Prioritizer
      | LD = LockDriver
      | PosW = PositionWindow
      | WL = WindowLogic
      | OW = ObstacleWindow
      | CWXC = ControlWindowXCentralized
      | S = Sensor
      | L = Lock
      | WPos = WindowPosition
      | M = Memory
      | InW = InputWindow
      | WIn = WindowInput
  PosW1 : Inport
  PosW2 : Inport  Port=2
  PosW4 : Inport  Port=3
  DW1 : Inport  Port=4
  DW2 : Inport  Port=5
  DW4 : Inport  Port=6
  P1W2 : Inport  Port=7
  P3W4 : Inport  Port=8
  P1W4 : Inport  Port=9
  OW1 : Inport  Port=10
  OW2 : Inport  Port=11
  OW4 : Inport  Port=12
  LD : Inport  Port=13
  CW1C : Inport  Port=14
  CW2C : Inport  Port=15
  CW4C : Inport  Port=16
  Pri : Subsystem
  Pri3 : Subsystem
  Pri4 : Subsystem
  WL : Subsystem
  WL1 : Subsystem
  WL3 : Subsystem
  W1 : Outport
  W2 : Outport  Port=2
  W4 : Outport  Port=3
  wires:
  CW4C/1 -> Pri4/4(CW4C)
  CW2C/1 -> Pri/3(CW2C)
  CW1C/1 -> Pri3/2(CW1C)
  Pri3/1(User) -> WL/2(User)
  WL3/1(WindowLogicOutput) -> W4/1
  Pri4/1(User) -> WL3/2(User)
  OW4/1 -> WL3/3(OW)
  PosW4/1 -> WL3/1(WPos)
  P1W4/1 -> Pri4/3(P1)
  P3W4/1 -> Pri4/2(P)
  DW4/1 -> Pri4/1(D)
  WL1/1(WindowLogicOutput) -> W2/1
  OW2/1 -> WL1/3(OW)
  PosW2/1 -> WL1/1(WPos)
  P1W2/1 -> Pri/2(P)
  DW2/1 -> Pri/1(D)
  Pri/1(User) -> WL1/2(User)
  WL/1(WindowLogicOutput) -> W1/1
  DW1/1 -> Pri3/1(D)
  OW1/1 -> WL/3(OW)
  PosW1/1 -> WL/1(WPos)
  LD/1 -> WL1/4(L), WL3/4(L), WL/4(L)

== system c00014M_harness/M034/Physical ==
  InW1 : Inport
  InW2 : Inport  Port=2
  InW4 : Inport  Port=3
  W : Subsystem
  W5 : Subsystem
  W7 : Subsystem
  W1 : Outport
  W2 : Outport  Port=2
  W4 : Outport  Port=3
  wires:
  W7/1(WPos) -> W4/1
  W5/1(WPos) -> W2/1
  W/1(WPos) -> W1/1
  InW4/1 -> W7/1(WIn)
  InW2/1 -> W5/1(WIn)
  InW1/1 -> W/1(WIn)

== system c00014M_harness/M034/S1 ==
  PhyMeasure : Inport
  SensorOut : Outport
  wires:
  PhyMeasure/1 -> SensorOut/1

== system c00014M_harness/M034/S2 ==
  PhyMeasure : Inport
  SensorOut : Outport
  wires:
  PhyMeasure/1 -> SensorOut/1

== system c00014M_harness/M034/S4 ==
  PhyMeasure : Inport
  SensorOut : Outport
  wires:
  PhyMeasure/1 -> SensorOut/1

== system c00014M_harness/M035/Cyber ==
  note: Sensors
  note: Inputs For Window1
  note: Inputs for Window 2
  note: Inputs for window 3
  note: Inputs for window 4
  note: Users
  note: Users
  note: Sensors
  note: Users
  note: Sensors
  note: Users
  note: Sensors
  note: USERS
      | ---------------------------------
      | 0: None
      | 1: Ventana Arriba
      | 2: Ventana hasta arriba
      | 3: Ventana abajo
      | 4: Ventana hasta abajo
  note: 1: SUBE
      | 0: PARADO
      | -1 BAJA
  note: D = Driver (W1)
      | P1 = Passenger 1 (W2)
      | P2 = Passenger 2 (W3)
      | P3 = Passenger 3 (W4)
      | O = Obstacle
      | C = Control
      | Pri = Prioritizer
      | LD = LockDriver
      | PosW = PositionWindow
      | WL = WindowLogic
      | OW = ObstacleWindow
      | CWXC = ControlWindowXCentralized
      | S = Sensor
      | L = Lock
      | WPos = WindowPosition
      | M = Memory
      | InW = InputWindow
      | WIn = WindowInput
  PosW1 : Inport
  PosW2 : Inport  Port=2
  PosW4 : Inport  Port=3
  DW1 : Inport  Port=4
  DW2 : Inport  Port=5
  DW4 : Inport  Port=6
  P1W2 : Inport  Port=7
  P3W4 : Inport  Port=8
  P1W4 : Inport  Port=9
  OW1 : Inport  Port=10
  OW2 : Inport  Port=11
  OW4 : Inport  Port=12
  LD : Inport  Port=13
  CW1C : Inport  Port=14
  CW2C : Inport  Port=15
  CW4C : Inport  Port=16
  Pri : Subsystem
  Pri3 : Subsystem
  Pri4 : Subsystem
  WL : Subsystem
  WL1 : Subsystem
  WL3 : Subsystem
  W1 : Outport
  W2 : Outport  Port=2
  W4 : Outport  Port=3
  wires:
  CW4C/1 -> Pri4/4(CW4C)
  CW2C/1 -> Pri/3(CW2C)
  CW1C/1 -> Pri3/2(CW1C)
  Pri3/1(User) -> WL/2(User)
  WL3/1(WindowLogicOutput) -> W4/1
  Pri4/1(User) -> WL3/2(User)
  OW4/1 -> WL3/3(OW)
  PosW4/1 -> WL3/1(WPos)
  P1W4/1 -> Pri4/3(P1)
  P3W4/1 -> Pri4/2(P)
  DW4/1 -> Pri4/1(D)
  WL1/1(WindowLogicOutput) -> W2/1
  OW2/1 -> WL1/3(OW)
  PosW2/1 -> WL1/1(WPos)
  P1W2/1 -> Pri/2(P)
  DW2/1 -> Pri/1(D)
  Pri/1(User) -> WL1/2(User)
  WL/1(WindowLogicOutput) -> W1/1
  DW1/1 -> Pri3/1(D)
  OW1/1 -> WL/3(OW)
  PosW1/1 -> WL/1(WPos)
  LD/1 -> WL1/4(L), WL3/4(L), WL/4(L)

== system c00014M_harness/M035/Physical ==
  InW1 : Inport
  InW2 : Inport  Port=2
  InW4 : Inport  Port=3
  W : Subsystem
  W5 : Subsystem
  W7 : Subsystem
  W1 : Outport
  W2 : Outport  Port=2
  W4 : Outport  Port=3
  wires:
  W7/1(WPos) -> W4/1
  W5/1(WPos) -> W2/1
  W/1(WPos) -> W1/1
  InW4/1 -> W7/1(WIn)
  InW2/1 -> W5/1(WIn)
  InW1/1 -> W/1(WIn)

== system c00014M_harness/M035/S1 ==
  PhyMeasure : Inport
  SensorOut : Outport
  wires:
  PhyMeasure/1 -> SensorOut/1

== system c00014M_harness/M035/S2 ==
  PhyMeasure : Inport
  SensorOut : Outport
  wires:
  PhyMeasure/1 -> SensorOut/1

== system c00014M_harness/M035/S4 ==
  PhyMeasure : Inport
  SensorOut : Outport
  wires:
  PhyMeasure/1 -> SensorOut/1

== system c00014M_harness/M036/Cyber ==
  note: Sensors
  note: Inputs For Window1
  note: Inputs for Window 2
  note: Inputs for window 3
  note: Inputs for window 4
  note: Users
  note: Users
  note: Sensors
  note: Users
  note: Sensors
  note: Users
  note: Sensors
  note: USERS
      | ---------------------------------
      | 0: None
      | 1: Ventana Arriba
      | 2: Ventana hasta arriba
      | 3: Ventana abajo
      | 4: Ventana hasta abajo
  note: 1: SUBE
      | 0: PARADO
      | -1 BAJA
  note: D = Driver (W1)
      | P1 = Passenger 1 (W2)
      | P2 = Passenger 2 (W3)
      | P3 = Passenger 3 (W4)
      | O = Obstacle
      | C = Control
      | Pri = Prioritizer
      | LD = LockDriver
      | PosW = PositionWindow
      | WL = WindowLogic
      | OW = ObstacleWindow
      | CWXC = ControlWindowXCentralized
      | S = Sensor
      | L = Lock
      | WPos = WindowPosition
      | M = Memory
      | InW = InputWindow
      | WIn = WindowInput
  PosW1 : Inport
  PosW2 : Inport  Port=2
  PosW4 : Inport  Port=3
  DW1 : Inport  Port=4
  DW2 : Inport  Port=5
  DW4 : Inport  Port=6
  P1W2 : Inport  Port=7
  P3W4 : Inport  Port=8
  P1W4 : Inport  Port=9
  OW1 : Inport  Port=10
  OW2 : Inport  Port=11
  OW4 : Inport  Port=12
  LD : Inport  Port=13
  CW1C : Inport  Port=14
  CW2C : Inport  Port=15
  CW4C : Inport  Port=16
  Pri : Subsystem
  Pri3 : Subsystem
  Pri4 : Subsystem
  WL : Subsystem
  WL1 : Subsystem
  WL3 : Subsystem
  W1 : Outport
  W2 : Outport  Port=2
  W4 : Outport  Port=3
  wires:
  CW4C/1 -> Pri4/4(CW4C)
  CW2C/1 -> Pri/3(CW2C)
  CW1C/1 -> Pri3/2(CW1C)
  Pri3/1(User) -> WL/2(User)
  WL3/1(WindowLogicOutput) -> W4/1
  Pri4/1(User) -> WL3/2(User)
  OW4/1 -> WL3/3(OW)
  PosW4/1 -> WL3/1(WPos)
  P1W4/1 -> Pri4/3(P1)
  P3W4/1 -> Pri4/2(P)
  DW4/1 -> Pri4/1(D)
  WL1/1(WindowLogicOutput) -> W2/1
  OW2/1 -> WL1/3(OW)
  PosW2/1 -> WL1/1(WPos)
  P1W2/1 -> Pri/2(P)
  DW2/1 -> Pri/1(D)
  Pri/1(User) -> WL1/2(User)
  WL/1(WindowLogicOutput) -> W1/1
  DW1/1 -> Pri3/1(D)
  OW1/1 -> WL/3(OW)
  PosW1/1 -> WL/1(WPos)
  LD/1 -> WL1/4(L), WL3/4(L), WL/4(L)

== system c00014M_harness/M036/Physical ==
  InW1 : Inport
  InW2 : Inport  Port=2
  InW4 : Inport  Port=3
  W : Subsystem
  W5 : Subsystem
  W7 : Subsystem
  W1 : Outport
  W2 : Outport  Port=2
  W4 : Outport  Port=3
  wires:
  W7/1(WPos) -> W4/1
  W5/1(WPos) -> W2/1
  W/1(WPos) -> W1/1
  InW4/1 -> W7/1(WIn)
  InW2/1 -> W5/1(WIn)
  InW1/1 -> W/1(WIn)

== system c00014M_harness/M036/S1 ==
  PhyMeasure : Inport
  SensorOut : Outport
  wires:
  PhyMeasure/1 -> SensorOut/1

== system c00014M_harness/M036/S2 ==
  PhyMeasure : Inport
  SensorOut : Outport
  wires:
  PhyMeasure/1 -> SensorOut/1

== system c00014M_harness/M036/S4 ==
  PhyMeasure : Inport
  SensorOut : Outport
  wires:
  PhyMeasure/1 -> SensorOut/1

== system c00014M_harness/M038/Cyber ==
  note: Sensors
  note: Inputs For Window1
  note: Inputs for Window 2
  note: Inputs for window 3
  note: Inputs for window 4
  note: Users
  note: Users
  note: Sensors
  note: Users
  note: Sensors
  note: Users
  note: Sensors
  note: USERS
      | ---------------------------------
      | 0: None
      | 1: Ventana Arriba
      | 2: Ventana hasta arriba
      | 3: Ventana abajo
      | 4: Ventana hasta abajo
  note: 1: SUBE
      | 0: PARADO
      | -1 BAJA
  note: D = Driver (W1)
      | P1 = Passenger 1 (W2)
      | P2 = Passenger 2 (W3)
      | P3 = Passenger 3 (W4)
      | O = Obstacle
      | C = Control
      | Pri = Prioritizer
      | LD = LockDriver
      | PosW = PositionWindow
      | WL = WindowLogic
      | OW = ObstacleWindow
      | CWXC = ControlWindowXCentralized
      | S = Sensor
      | L = Lock
      | WPos = WindowPosition
      | M = Memory
      | InW = InputWindow
      | WIn = WindowInput
  PosW1 : Inport
  PosW2 : Inport  Port=2
  PosW4 : Inport  Port=3
  DW1 : Inport  Port=4
  DW2 : Inport  Port=5
  DW4 : Inport  Port=6
  P1W2 : Inport  Port=7
  P3W4 : Inport  Port=8
  P1W4 : Inport  Port=9
  OW1 : Inport  Port=10
  OW2 : Inport  Port=11
  OW4 : Inport  Port=12
  LD : Inport  Port=13
  CW1C : Inport  Port=14
  CW2C : Inport  Port=15
  CW4C : Inport  Port=16
  Pri : Subsystem
  Pri3 : Subsystem
  Pri4 : Subsystem
  WL : Subsystem
  WL1 : Subsystem
  WL3 : Subsystem
  W1 : Outport
  W2 : Outport  Port=2
  W4 : Outport  Port=3
  wires:
  CW4C/1 -> Pri4/4(CW4C)
  CW2C/1 -> Pri/3(CW2C)
  CW1C/1 -> Pri3/2(CW1C)
  Pri3/1(User) -> WL/2(User)
  WL3/1(WindowLogicOutput) -> W4/1
  Pri4/1(User) -> WL3/2(User)
  OW4/1 -> WL3/3(OW)
  PosW4/1 -> WL3/1(WPos)
  P1W4/1 -> Pri4/3(P1)
  P3W4/1 -> Pri4/2(P)
  DW4/1 -> Pri4/1(D)
  WL1/1(WindowLogicOutput) -> W2/1
  OW2/1 -> WL1/3(OW)
  PosW2/1 -> WL1/1(WPos)
  P1W2/1 -> Pri/2(P)
  DW2/1 -> Pri/1(D)
  Pri/1(User) -> WL1/2(User)
  WL/1(WindowLogicOutput) -> W1/1
  DW1/1 -> Pri3/1(D)
  OW1/1 -> WL/3(OW)
  PosW1/1 -> WL/1(WPos)
  LD/1 -> WL1/4(L), WL3/4(L), WL/4(L)

== system c00014M_harness/M038/Physical ==
  InW1 : Inport
  InW2 : Inport  Port=2
  InW4 : Inport  Port=3
  W : Subsystem
  W5 : Subsystem
  W7 : Subsystem
  W1 : Outport
  W2 : Outport  Port=2
  W4 : Outport  Port=3
  wires:
  W7/1(WPos) -> W4/1
  W5/1(WPos) -> W2/1
  W/1(WPos) -> W1/1
  InW4/1 -> W7/1(WIn)
  InW2/1 -> W5/1(WIn)
  InW1/1 -> W/1(WIn)

== system c00014M_harness/M038/S1 ==
  PhyMeasure : Inport
  SensorOut : Outport
  wires:
  PhyMeasure/1 -> SensorOut/1

== system c00014M_harness/M038/S2 ==
  PhyMeasure : Inport
  SensorOut : Outport
  wires:
  PhyMeasure/1 -> SensorOut/1

== system c00014M_harness/M038/S4 ==
  PhyMeasure : Inport
  SensorOut : Outport
  wires:
  PhyMeasure/1 -> SensorOut/1

== system c00014M_harness/M039/Cyber ==
  note: Sensors
  note: Inputs For Window1
  note: Inputs for Window 2
  note: Inputs for window 3
  note: Inputs for window 4
  note: Users
  note: Users
  note: Sensors
  note: Users
  note: Sensors
  note: Users
  note: Sensors
  note: USERS
      | ---------------------------------
      | 0: None
      | 1: Ventana Arriba
      | 2: Ventana hasta arriba
      | 3: Ventana abajo
      | 4: Ventana hasta abajo
  note: 1: SUBE
      | 0: PARADO
      | -1 BAJA
  note: D = Driver (W1)
      | P1 = Passenger 1 (W2)
      | P2 = Passenger 2 (W3)
      | P3 = Passenger 3 (W4)
      | O = Obstacle
      | C = Control
      | Pri = Prioritizer
      | LD = LockDriver
      | PosW = PositionWindow
      | WL = WindowLogic
      | OW = ObstacleWindow
      | CWXC = ControlWindowXCentralized
      | S = Sensor
      | L = Lock
      | WPos = WindowPosition
      | M = Memory
      | InW = InputWindow
      | WIn = WindowInput
  PosW1 : Inport
  PosW2 : Inport  Port=2
  PosW4 : Inport  Port=3
  DW1 : Inport  Port=4
  DW2 : Inport  Port=5
  DW4 : Inport  Port=6
  P1W2 : Inport  Port=7
  P3W4 : Inport  Port=8
  P1W4 : Inport  Port=9
  OW1 : Inport  Port=10
  OW2 : Inport  Port=11
  OW4 : Inport  Port=12
  LD : Inport  Port=13
  CW1C : Inport  Port=14
  CW2C : Inport  Port=15
  CW4C : Inport  Port=16
  Pri : Subsystem
  Pri3 : Subsystem
  Pri4 : Subsystem
  WL : Subsystem
  WL1 : Subsystem
  WL3 : Subsystem
  W1 : Outport
  W2 : Outport  Port=2
  W4 : Outport  Port=3
  wires:
  CW4C/1 -> Pri4/4(CW4C)
  CW2C/1 -> Pri/3(CW2C)
  CW1C/1 -> Pri3/2(CW1C)
  Pri3/1(User) -> WL/2(User)
  WL3/1(WindowLogicOutput) -> W4/1
  Pri4/1(User) -> WL3/2(User)
  OW4/1 -> WL3/3(OW)
  PosW4/1 -> WL3/1(WPos)
  P1W4/1 -> Pri4/3(P1)
  P3W4/1 -> Pri4/2(P)
  DW4/1 -> Pri4/1(D)
  WL1/1(WindowLogicOutput) -> W2/1
  OW2/1 -> WL1/3(OW)
  PosW2/1 -> WL1/1(WPos)
  P1W2/1 -> Pri/2(P)
  DW2/1 -> Pri/1(D)
  Pri/1(User) -> WL1/2(User)
  WL/1(WindowLogicOutput) -> W1/1
  DW1/1 -> Pri3/1(D)
  OW1/1 -> WL/3(OW)
  PosW1/1 -> WL/1(WPos)
  LD/1 -> WL1/4(L), WL3/4(L), WL/4(L)

== system c00014M_harness/M039/Physical ==
  InW1 : Inport
  InW2 : Inport  Port=2
  InW4 : Inport  Port=3
  W : Subsystem
  W5 : Subsystem
  W7 : Subsystem
  W1 : Outport
  W2 : Outport  Port=2
  W4 : Outport  Port=3
  wires:
  W7/1(WPos) -> W4/1
  W5/1(WPos) -> W2/1
  W/1(WPos) -> W1/1
  InW4/1 -> W7/1(WIn)
  InW2/1 -> W5/1(WIn)
  InW1/1 -> W/1(WIn)

== system c00014M_harness/M039/S1 ==
  PhyMeasure : Inport
  SensorOut : Outport
  wires:
  PhyMeasure/1 -> SensorOut/1

== system c00014M_harness/M039/S2 ==
  PhyMeasure : Inport
  SensorOut : Outport
  wires:
  PhyMeasure/1 -> SensorOut/1

== system c00014M_harness/M039/S4 ==
  PhyMeasure : Inport
  SensorOut : Outport
  wires:
  PhyMeasure/1 -> SensorOut/1

== system c00014M_harness/M040/Cyber ==
  note: Sensors
  note: Inputs For Window1
  note: Inputs for Window 2
  note: Inputs for window 3
  note: Inputs for window 4
  note: Users
  note: Users
  note: Sensors
  note: Users
  note: Sensors
  note: Users
  note: Sensors
  note: USERS
      | ---------------------------------
      | 0: None
      | 1: Ventana Arriba
      | 2: Ventana hasta arriba
      | 3: Ventana abajo
      | 4: Ventana hasta abajo
  note: 1: SUBE
      | 0: PARADO
      | -1 BAJA
  note: D = Driver (W1)
      | P1 = Passenger 1 (W2)
      | P2 = Passenger 2 (W3)
      | P3 = Passenger 3 (W4)
      | O = Obstacle
      | C = Control
      | Pri = Prioritizer
      | LD = LockDriver
      | PosW = PositionWindow
      | WL = WindowLogic
      | OW = ObstacleWindow
      | CWXC = ControlWindowXCentralized
      | S = Sensor
      | L = Lock
      | WPos = WindowPosition
      | M = Memory
      | InW = InputWindow
      | WIn = WindowInput
  PosW1 : Inport
  PosW2 : Inport  Port=2
  PosW4 : Inport  Port=3
  DW1 : Inport  Port=4
  DW2 : Inport  Port=5
  DW4 : Inport  Port=6
  P1W2 : Inport  Port=7
  P3W4 : Inport  Port=8
  P1W4 : Inport  Port=9
  OW1 : Inport  Port=10
  OW2 : Inport  Port=11
  OW4 : Inport  Port=12
  LD : Inport  Port=13
  CW1C : Inport  Port=14
  CW2C : Inport  Port=15
  CW4C : Inport  Port=16
  Pri : Subsystem
  Pri3 : Subsystem
  Pri4 : Subsystem
  WL : Subsystem
  WL1 : Subsystem
  WL3 : Subsystem
  W1 : Outport
  W2 : Outport  Port=2
  W4 : Outport  Port=3
  wires:
  CW4C/1 -> Pri4/4(CW4C)
  CW2C/1 -> Pri/3(CW2C)
  CW1C/1 -> Pri3/2(CW1C)
  Pri3/1(User) -> WL/2(User)
  WL3/1(WindowLogicOutput) -> W4/1
  Pri4/1(User) -> WL3/2(User)
  OW4/1 -> WL3/3(OW)
  PosW4/1 -> WL3/1(WPos)
  P1W4/1 -> Pri4/3(P1)
  P3W4/1 -> Pri4/2(P)
  DW4/1 -> Pri4/1(D)
  WL1/1(WindowLogicOutput) -> W2/1
  OW2/1 -> WL1/3(OW)
  PosW2/1 -> WL1/1(WPos)
  P1W2/1 -> Pri/2(P)
  DW2/1 -> Pri/1(D)
  Pri/1(User) -> WL1/2(User)
  WL/1(WindowLogicOutput) -> W1/1
  DW1/1 -> Pri3/1(D)
  OW1/1 -> WL/3(OW)
  PosW1/1 -> WL/1(WPos)
  LD/1 -> WL1/4(L), WL3/4(L), WL/4(L)

== system c00014M_harness/M040/Physical ==
  InW1 : Inport
  InW2 : Inport  Port=2
  InW4 : Inport  Port=3
  W : Subsystem
  W5 : Subsystem
  W7 : Subsystem
  W1 : Outport
  W2 : Outport  Port=2
  W4 : Outport  Port=3
  wires:
  W7/1(WPos) -> W4/1
  W5/1(WPos) -> W2/1
  W/1(WPos) -> W1/1
  InW4/1 -> W7/1(WIn)
  InW2/1 -> W5/1(WIn)
  InW1/1 -> W/1(WIn)

== system c00014M_harness/M040/S1 ==
  PhyMeasure : Inport
  SensorOut : Outport
  wires:
  PhyMeasure/1 -> SensorOut/1

== system c00014M_harness/M040/S2 ==
  PhyMeasure : Inport
  SensorOut : Outport
  wires:
  PhyMeasure/1 -> SensorOut/1

== system c00014M_harness/M040/S4 ==
  PhyMeasure : Inport
  SensorOut : Outport
  wires:
  PhyMeasure/1 -> SensorOut/1

== system c00014M_harness/M042/Cyber ==
  note: Sensors
  note: Inputs For Window1
  note: Inputs for Window 2
  note: Inputs for window 3
  note: Inputs for window 4
  note: Users
  note: Users
  note: Sensors
  note: Users
  note: Sensors
  note: Users
  note: Sensors
  note: USERS
      | ---------------------------------
      | 0: None
      | 1: Ventana Arriba
      | 2: Ventana hasta arriba
      | 3: Ventana abajo
      | 4: Ventana hasta abajo
  note: 1: SUBE
      | 0: PARADO
      | -1 BAJA
  note: D = Driver (W1)
      | P1 = Passenger 1 (W2)
      | P2 = Passenger 2 (W3)
      | P3 = Passenger 3 (W4)
      | O = Obstacle
      | C = Control
      | Pri = Prioritizer
      | LD = LockDriver
      | PosW = PositionWindow
      | WL = WindowLogic
      | OW = ObstacleWindow
      | CWXC = ControlWindowXCentralized
      | S = Sensor
      | L = Lock
      | WPos = WindowPosition
      | M = Memory
      | InW = InputWindow
      | WIn = WindowInput
  PosW1 : Inport
  PosW2 : Inport  Port=2
  PosW4 : Inport  Port=3
  DW1 : Inport  Port=4
  DW2 : Inport  Port=5
  DW4 : Inport  Port=6
  P1W2 : Inport  Port=7
  P3W4 : Inport  Port=8
  P1W4 : Inport  Port=9
  OW1 : Inport  Port=10
  OW2 : Inport  Port=11
  OW4 : Inport  Port=12
  LD : Inport  Port=13
  CW1C : Inport  Port=14
  CW2C : Inport  Port=15
  CW4C : Inport  Port=16
  Pri : Subsystem
  Pri3 : Subsystem
  Pri4 : Subsystem
  WL : Subsystem
  WL1 : Subsystem
  WL3 : Subsystem
  W1 : Outport
  W2 : Outport  Port=2
  W4 : Outport  Port=3
  wires:
  CW4C/1 -> Pri4/4(CW4C)
  CW2C/1 -> Pri/3(CW2C)
  CW1C/1 -> Pri3/2(CW1C)
  Pri3/1(User) -> WL/2(User)
  WL3/1(WindowLogicOutput) -> W4/1
  Pri4/1(User) -> WL3/2(User)
  OW4/1 -> WL3/3(OW)
  PosW4/1 -> WL3/1(WPos)
  P1W4/1 -> Pri4/3(P1)
  P3W4/1 -> Pri4/2(P)
  DW4/1 -> Pri4/1(D)
  WL1/1(WindowLogicOutput) -> W2/1
  OW2/1 -> WL1/3(OW)
  PosW2/1 -> WL1/1(WPos)
  P1W2/1 -> Pri/2(P)
  DW2/1 -> Pri/1(D)
  Pri/1(User) -> WL1/2(User)
  WL/1(WindowLogicOutput) -> W1/1
  DW1/1 -> Pri3/1(D)
  OW1/1 -> WL/3(OW)
  PosW1/1 -> WL/1(WPos)
  LD/1 -> WL1/4(L), WL3/4(L), WL/4(L)

== system c00014M_harness/M042/Physical ==
  InW1 : Inport
  InW2 : Inport  Port=2
  InW4 : Inport  Port=3
  W : Subsystem
  W5 : Subsystem
  W7 : Subsystem
  W1 : Outport
  W2 : Outport  Port=2
  W4 : Outport  Port=3
  wires:
  W7/1(WPos) -> W4/1
  W5/1(WPos) -> W2/1
  W/1(WPos) -> W1/1
  InW4/1 -> W7/1(WIn)
  InW2/1 -> W5/1(WIn)
  InW1/1 -> W/1(WIn)

== system c00014M_harness/M042/S1 ==
  PhyMeasure : Inport
  SensorOut : Outport
  wires:
  PhyMeasure/1 -> SensorOut/1

== system c00014M_harness/M042/S2 ==
  PhyMeasure : Inport
  SensorOut : Outport
  wires:
  PhyMeasure/1 -> SensorOut/1

== system c00014M_harness/M042/S4 ==
  PhyMeasure : Inport
  SensorOut : Outport
  wires:
  PhyMeasure/1 -> SensorOut/1
